simulink model "sdm_sec"  (Simulink 8.1)
settings: Solver=ode45  StartTime=0.0  StopTime=10.0  RelTol=1e-3
undefined symbols (not defined in the file or in its folder): qunt, qunt1
settings Model: Creator=amr  LastModifiedBy=amr
settings DataIOCC: SignalLoggingSaveFormat=Dataset
settings OptimizationCC: ExpressionDepthLimit=128
settings DebuggingCC: FcnCallInpInsideContextMsg=EnableAllAsError
settings GRTTargetCC: CombineOutputUpdateFcns=on  GRTInterface=off

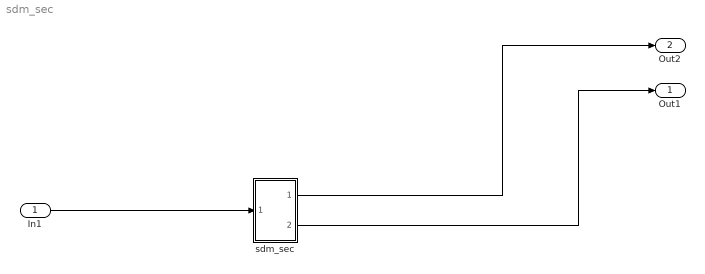
== system sdm_sec ==
  In1 : Inport
  sdm_sec : Subsystem
  Out1 : Outport
  Out2 : Outport  Port=2
  wires:
  In1/1 -> sdm_sec/1(In1)
  sdm_sec/1(dout) -> Out2/1
  sdm_sec/2(qunt_out) -> Out1/1

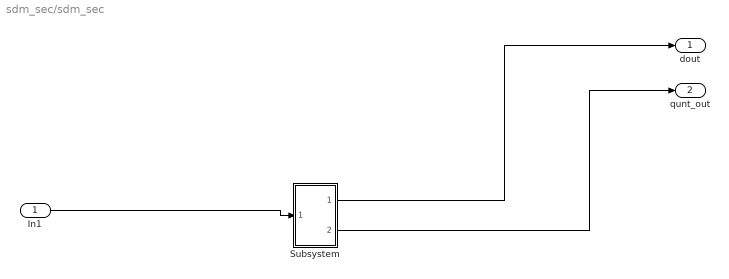
== system sdm_sec/sdm_sec ==
  In1 : Inport
  Subsystem : Subsystem
  dout : Outport
  qunt_out : Outport  Port=2
  wires:
  In1/1 -> Subsystem/1(In1)
  Subsystem/1(Out1) -> dout/1
  Subsystem/2(Out2) -> qunt_out/1

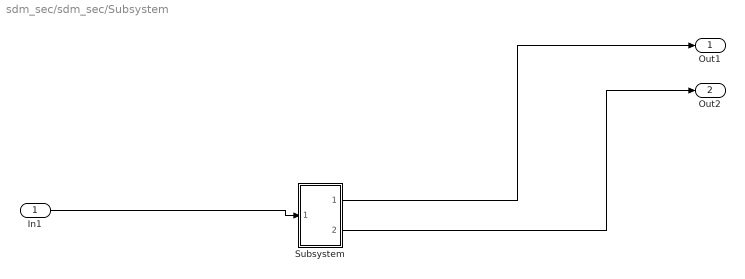
== system sdm_sec/sdm_sec/Subsystem ==
  In1 : Inport
  Subsystem : Subsystem
  Out1 : Outport
  Out2 : Outport  Port=2
  wires:
  In1/1 -> Subsystem/1(In1)
  Subsystem/1(Out1) -> Out1/1
  Subsystem/2(Out2) -> Out2/1

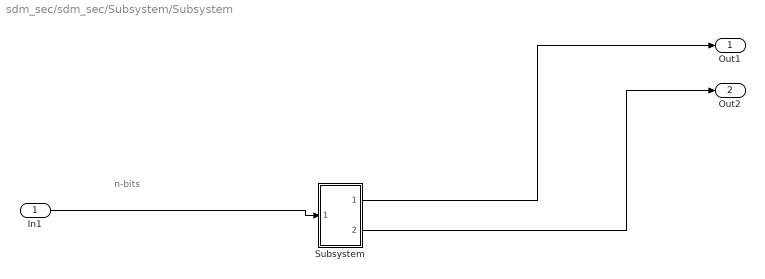
== system sdm_sec/sdm_sec/Subsystem/Subsystem ==
  note: n-bits
  In1 : Inport
  Subsystem : Subsystem
  Out1 : Outport
  Out2 : Outport  Port=2
  wires:
  In1/1 -> Subsystem/1(In1)
  Subsystem/1(Out1) -> Out1/1
  Subsystem/2(Out2) -> Out2/1

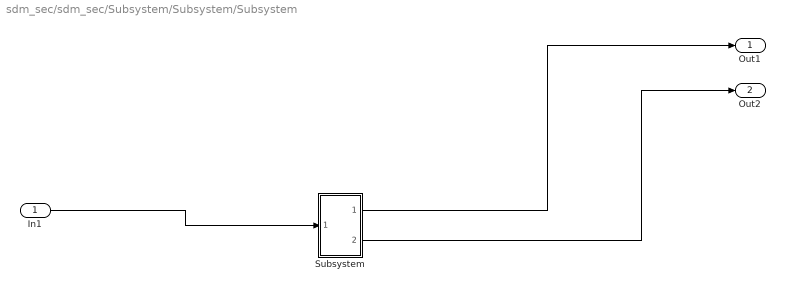
== system sdm_sec/sdm_sec/Subsystem/Subsystem/Subsystem ==
  In1 : Inport
  Subsystem : Subsystem
  Out1 : Outport
  Out2 : Outport  Port=2
  wires:
  In1/1 -> Subsystem/1(In1)
  Subsystem/1(Out1) -> Out1/1
  Subsystem/2(Out2) -> Out2/1

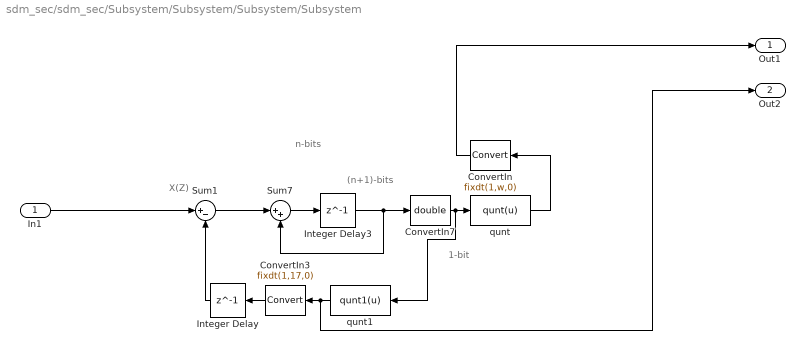
== system sdm_sec/sdm_sec/Subsystem/Subsystem/Subsystem/Subsystem ==
  note: X(Z)
  note: 1-bit
  note: (n+1)-bits
  note: n-bits
  In1 : Inport
  ConvertIn : DataTypeConversion  OutDataTypeStr=fixdt(1,w,0)
  ConvertIn3 : DataTypeConversion  OutDataTypeStr=fixdt(1,17,0)
  ConvertIn7 : DataTypeConversion  OutDataTypeStr=double
  Integer Delay : Delay  DelayLength=1  InputProcessing=Inherited
  Integer Delay3 : Delay  DelayLength=1  InputProcessing=Inherited
  Sum1 : Sum  Inputs=|+-  OutDataTypeStr=fixdt(1,w,0)
  Sum7 : Sum  Inputs=|++  OutDataTypeStr=fixdt(1,w+1,0)
  qunt : MATLABFcn  MATLABFcn=qunt(u)  OutputDimensions=1
  qunt1 : MATLABFcn  MATLABFcn=qunt1(u)  OutputDimensions=1
  Out1 : Outport
  Out2 : Outport  Port=2
  wires:
  qunt1/1 -> Out2/1, ConvertIn3/1
  Sum7/1 -> Integer Delay3/1
  qunt/1 -> ConvertIn/1
  ConvertIn7/1 -> qunt1/1, qunt/1
  Integer Delay/1 -> Sum1/2
  ConvertIn/1 -> Out1/1
  ConvertIn3/1 -> Integer Delay/1
  Sum1/1 -> Sum7/1
  In1/1 -> Sum1/1
  Integer Delay3/1 -> Sum7/2, ConvertIn7/1
